simulink model "Path_Planner"  (R2023b)
settings: Solver=FixedStepDiscrete  StartTime=0.0  StopTime=inf  FixedStep=0.010  RelTol=1e-3
settings Model: Creator=Darsh  LastModifiedBy=Darsh
settings RTWCC: Description=Generate an RTMaps component embedding the model  SystemTargetFile=rtmaps.tlc  TemplateMakefile=rtmaps_default_tmf  PostCodeGenCommand=rtmaps_post_code_generation(buildInfo)  RetainRTWFile=on  TargetLang=C++
settings STFCustomTargetCC: TargetLangStandard=C++11 (ISO)  ModelReferenceCompliant=off  CombineOutputUpdateFcns=on  SystemTargetFile=rtmaps.tlc
settings GRTTargetCC: TargetLangStandard=C++11 (ISO)  ModelReferenceCompliant=off  ParMdlRefBuildCompliant=off  CompOptLevelCompliant=off  ConcurrentExecutionCompliant=off  MatFileLogging=off  CPPClassGenCompliant=off  UseToolchainInfoCompliant=off

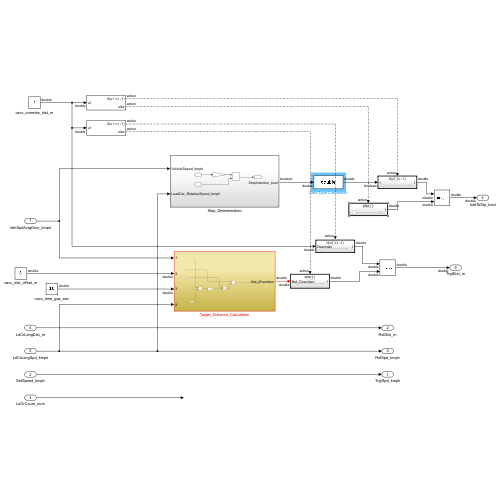
[thumbnail: Simulink's stored preview of the top-level diagram]
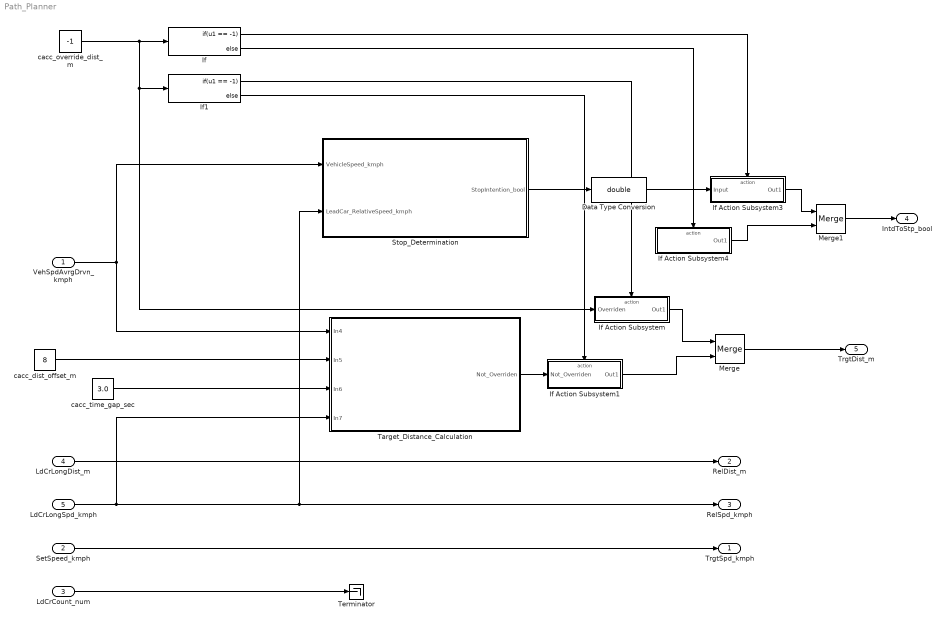
== system Path_Planner ==
  VehSpdAvrgDrvn_kmph : Inport
  SetSpeed_kmph : Inport  Port=2
  LdCrCount_num : Inport  Port=3
  LdCrLongDist_m : Inport  Port=4
  LdCrLongSpd_kmph : Inport  Port=5
  Data Type Conversion : DataTypeConversion  OutDataTypeStr=double  SaturateOnIntegerOverflow=off  RndMeth=Floor
  If : If  IfExpression=u1 == -1
  If Action Subsystem : Subsystem  TreatAsAtomicUnit=on
  If Action Subsystem1 : Subsystem  TreatAsAtomicUnit=on
  If Action Subsystem3 : Subsystem  TreatAsAtomicUnit=on
  If Action Subsystem4 : Subsystem  TreatAsAtomicUnit=on
  If1 : If  IfExpression=u1 == -1
  Merge : Merge
  Merge1 : Merge
  Stop_Determination : Subsystem
  Target_Distance_Calculation : Subsystem
  Terminator : Terminator
  cacc_dist_offset_m : Constant  Value=8
  cacc_override_dist_m : Constant  Value=-1
  cacc_time_gap_sec : Constant  Value=3.0
  TrgtSpd_kmph : Outport
  RelDist_m : Outport  Port=2
  RelSpd_kmph : Outport  Port=3
  IntdToStp_bool : Outport  Port=4
  TrgtDist_m : Outport  Port=5
  wires:
  SetSpeed_kmph/1 -> TrgtSpd_kmph/1
  LdCrLongSpd_kmph/1 -> Target_Distance_Calculation/4(In7), RelSpd_kmph/1, Stop_Determination/2(LeadCar_RelativeSpeed_kmph)
  LdCrLongDist_m/1 -> RelDist_m/1
  LdCrCount_num/1 -> Terminator/1
  cacc_dist_offset_m/1 -> Target_Distance_Calculation/2(In5)
  cacc_time_gap_sec/1 -> Target_Distance_Calculation/3(In6)
  If/2 -> If Action Subsystem4/Action
  If/1 -> If Action Subsystem3/Action
  If Action Subsystem/1(Out1) -> Merge/1
  Merge/1 -> TrgtDist_m/1
  If Action Subsystem1/1(Out1) -> Merge/2
  cacc_override_dist_m/1 -> If/1, If1/1, If Action Subsystem/1(Overriden)
  If Action Subsystem4/1(Out1) -> Merge1/2
  If Action Subsystem3/1(Out1) -> Merge1/1
  Merge1/1 -> IntdToStp_bool/1
  Stop_Determination/1(StopIntention_bool) -> Data Type Conversion/1
  Target_Distance_Calculation/1(Not_Overriden) -> If Action Subsystem1/1(Not_Overriden)
  VehSpdAvrgDrvn_kmph/1 -> Target_Distance_Calculation/1(In4), Stop_Determination/1(VehicleSpeed_kmph)
  If1/1 -> If Action Subsystem/Action
  If1/2 -> If Action Subsystem1/Action
  Data Type Conversion/1 -> If Action Subsystem3/1(Input)

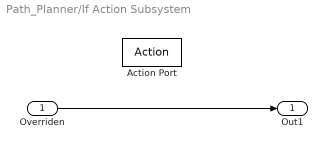
== system Path_Planner/If Action Subsystem ==
  Overriden : Inport
  Action Port : ActionPort  ActionPortLabel=if(u1 == -1)
  Out1 : Outport
  wires:
  Overriden/1 -> Out1/1

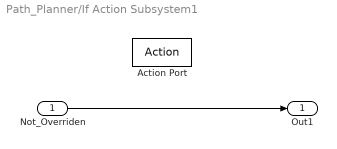
== system Path_Planner/If Action Subsystem1 ==
  Not_Overriden : Inport
  Action Port : ActionPort  ActionPortLabel=else
  Out1 : Outport
  wires:
  Not_Overriden/1 -> Out1/1

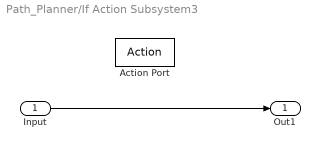
== system Path_Planner/If Action Subsystem3 ==
  Input : Inport
  Action Port : ActionPort  ActionPortLabel=if(u1 == -1)
  Out1 : Outport
  wires:
  Input/1 -> Out1/1

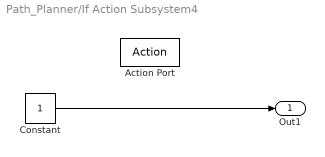
== system Path_Planner/If Action Subsystem4 ==
  Action Port : ActionPort  ActionPortLabel=else
  Constant : Constant
  Out1 : Outport
  wires:
  Constant/1 -> Out1/1

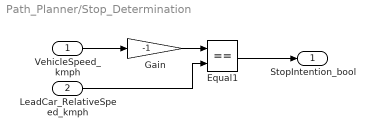
== system Path_Planner/Stop_Determination ==
  VehicleSpeed_kmph : Inport
  LeadCar_RelativeSpeed_kmph : Inport  Port=2
  Equal1 : RelationalOperator  Operator===  OutDataTypeStr=boolean  RndMeth=Simplest  InputSameDT=off
  Gain : Gain  Gain=-1
  StopIntention_bool : Outport
  wires:
  Gain/1 -> Equal1/1
  VehicleSpeed_kmph/1 -> Gain/1
  LeadCar_RelativeSpeed_kmph/1 -> Equal1/2
  Equal1/1 -> StopIntention_bool/1

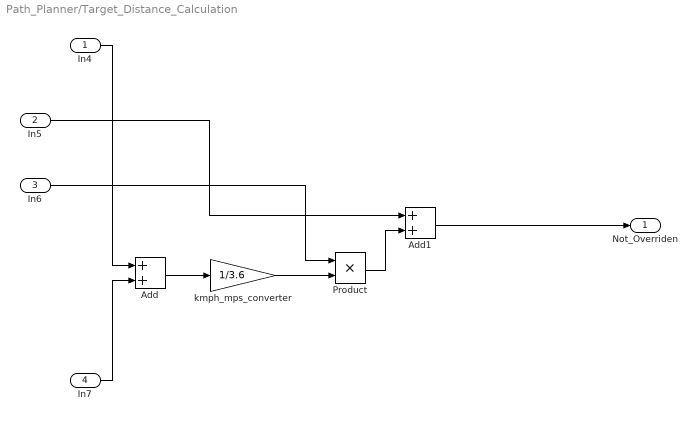
== system Path_Planner/Target_Distance_Calculation ==
  In4 : Inport
  In5 : Inport  Port=2
  In6 : Inport  Port=3
  In7 : Inport  Port=4
  Add : Sum
  Add1 : Sum
  Product : Product
  kmph_mps_converter : Gain  Gain=1/3.6
  Not_Overriden : Outport
  wires:
  Add/1 -> kmph_mps_converter/1
  Product/1 -> Add1/2
  kmph_mps_converter/1 -> Product/2
  In4/1 -> Add/1
  In7/1 -> Add/2
  In6/1 -> Product/1
  In5/1 -> Add1/1
  Add1/1 -> Not_Overriden/1
